simulink model "HighwayLaneChangePlanner"  (R2024b)
settings: Solver=FixedStepAuto  StartTime=0.0  StopTime=10.0  RelTol=1e-3  EnableMultiTasking=on
undefined symbols (not defined in the file or in its folder): actorProfiles, Ts
(part 1 of 2)
settings Model: Creator=The MathWorks, Inc.  LastModifiedBy=grape4314
settings SolverCC: AlgebraicLoopSolver=TrustRegion  MaxZcPerStep=1
settings DataIOCC: SaveOutput=off
settings OptimizationCC: DefaultParameterBehavior=Inlined  InlineInvariantSignals=on  EnhancedBackFolding=on  PassReuseOutputArgsAs=Individual arguments  ZeroExternalMemoryAtStartup=off  ZeroInternalMemoryAtStartup=off  EfficientFloat2IntCast=on  OptimizeBlockOrder=speed  DifferentSizesBufferReuse=on  OptimizationCustomize=off  EfficientTunableParamExpr=on
settings DebuggingCC: ParameterTunabilityLossMsg=error  UnconnectedInputMsg=warning  UnconnectedOutputMsg=warning  UnconnectedLineMsg=warning  ModelReferenceSymbolNameMessage=none  SubsystemReferenceDiagnosticForUnitTest=warning
settings HardwareCC: ProdLongLongMode=on
settings ModelReferenceCC: EnableRefExpFcnMdlSchedulingChecks=on  ModelReferenceNumInstancesAllowed=Single  PropagateVarSize=During execution
settings RTWCC: Description=Embedded Coder  SystemTargetFile=ert.tlc  TemplateMakefile=ert_default_tmf  RTWVerbose=off  BuildConfiguration=Faster Runs  PortableWordSizes=on  CodeExecutionProfiling=on  CodeProfilingSaveOptions=AllData  TargetLang=C++  GPUComputeCapability=3.5  DLArmComputeVersion=19.05
settings CodeAppCC: ForceParamTrailComments=on  IgnoreCustomStorageClasses=off  OperatorAnnotations=on  SimulinkDataObjDesc=on  SFDataObjDesc=on  CustomSymbolStrGlobalVar=$N$M  CustomSymbolStrType=$N$M_T  CustomSymbolStrFcn=APV_$N$M$F  CustomSymbolStrMacro=$N$M  InsertBlockDesc=on
settings ERTTargetCC: TargetLangStandard=C++03 (ISO)  GenerateSampleERTMain=on  CombineSignalStateStructs=on  CodeInterfacePackaging=C++ class  SupportVariableSizeSignals=on  RootIOFormat=Structure reference  ERTCustomFileTemplate=example_file_process.tlc  DynamicArrayContainerType=coder::array

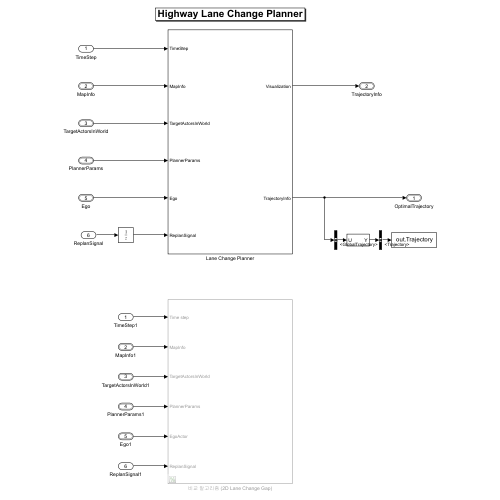
[thumbnail: Simulink's stored preview of the top-level diagram]
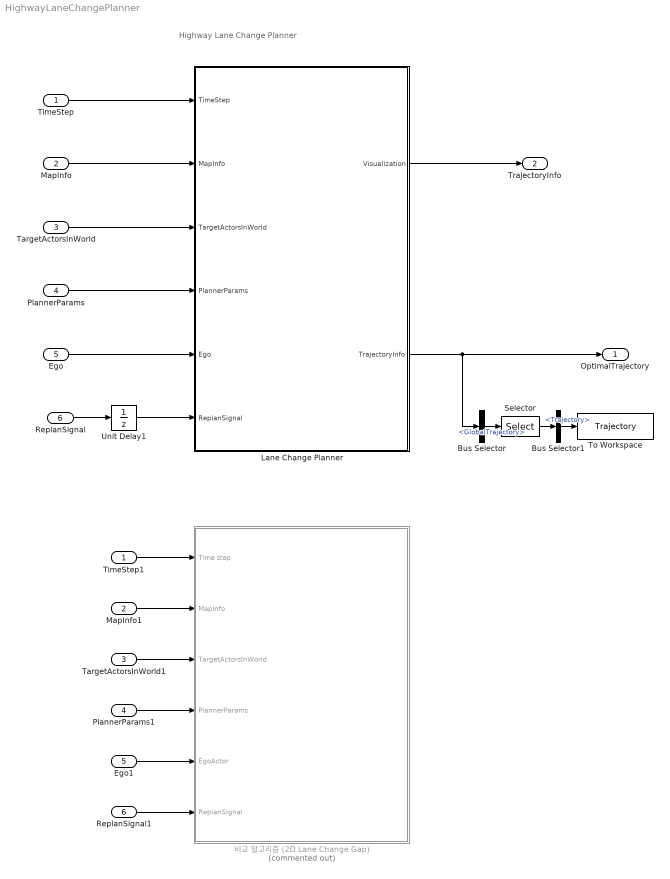
== system HighwayLaneChangePlanner ==
  note: Highway Lane Change Planner
  TimeStep : Inport
  MapInfo : Inport  Port=2  OutDataTypeStr=Bus: BusMapInfo  BusOutputAsStruct=on
  TargetActorsInWorld : Inport  Port=3  OutDataTypeStr=Bus: BusActorsEgo  BusOutputAsStruct=on
  PlannerParams : Inport  Port=4  OutDataTypeStr=Bus: BusPlannerParams  BusOutputAsStruct=on
  Ego : Inport  Port=5  OutDataTypeStr=Bus: BusVehiclePose
  ReplanSignal : Inport  Port=6
  Bus Selector : BusSelector  OutputSignals=GlobalTrajectory
  Bus Selector1 : BusSelector  OutputSignals=Trajectory
  Ego1 : InportShadow  Port=5  OutDataTypeStr=Bus: BusVehiclePose
  Lane Change Planner : Subsystem
  MapInfo1 : InportShadow  Port=2  OutDataTypeStr=Bus: BusMapInfo  BusOutputAsStruct=on
  PlannerParams1 : InportShadow  Port=4  OutDataTypeStr=Bus: BusPlannerParams  BusOutputAsStruct=on
  ReplanSignal1 : InportShadow  Port=6
  Selector : Selector  InputPortWidth=30  IndexOptions=Index vector (dialog)  Indices=1  OutputSizes=1
  TargetActorsInWorld1 : InportShadow  Port=3  OutDataTypeStr=Bus: BusActorsEgo  BusOutputAsStruct=on
  TimeStep1 : InportShadow
  To Workspace : ToWorkspace  VariableName=Trajectory  SaveFormat=Structure With Time  SampleTime=-1
  Unit Delay1 : UnitDelay  InitialCondition=1  SampleTime=-1  HasFrameUpgradeWarning=on
  비교 알고리즘 (2D Lane Change Gap) : Subsystem  Commented=on
  OptimalTrajectory : Outport  OutDataTypeStr=Bus: BusGlobalTrajectories  BusOutputAsStruct=on
  TrajectoryInfo : Outport  Port=2  OutDataTypeStr=Bus: BusVisualizationInfo  BusOutputAsStruct=on
  wires:
  TimeStep/1 -> Lane Change Planner/1(TimeStep)
  MapInfo/1 -> Lane Change Planner/2(MapInfo)
  TargetActorsInWorld/1 -> Lane Change Planner/3(TargetActorsInWorld)
  PlannerParams/1 -> Lane Change Planner/4(PlannerParams)
  Ego/1 -> Lane Change Planner/5(Ego)
  Lane Change Planner/1(Visualization) -> TrajectoryInfo/1
  Lane Change Planner/2(TrajectoryInfo) -> Bus Selector/1, OptimalTrajectory/1
  ReplanSignal/1 -> Unit Delay1/1
  Unit Delay1/1 -> Lane Change Planner/6(ReplanSignal)
  TimeStep1/1 -> 비교 알고리즘 (2D Lane Change Gap)/1(Time step)
  MapInfo1/1 -> 비교 알고리즘 (2D Lane Change Gap)/2(MapInfo)
  TargetActorsInWorld1/1 -> 비교 알고리즘 (2D Lane Change Gap)/3(TargetActorsInWorld)
  PlannerParams1/1 -> 비교 알고리즘 (2D Lane Change Gap)/4(PlannerParams)
  Ego1/1 -> 비교 알고리즘 (2D Lane Change Gap)/5(EgoActor)
  ReplanSignal1/1 -> 비교 알고리즘 (2D Lane Change Gap)/6(ReplanSignal)
  Bus Selector/1 -> Selector/1  "<GlobalTrajectory>"
  Bus Selector1/1 -> To Workspace/1  "<Trajectory>"
  Selector/1 -> Bus Selector1/1

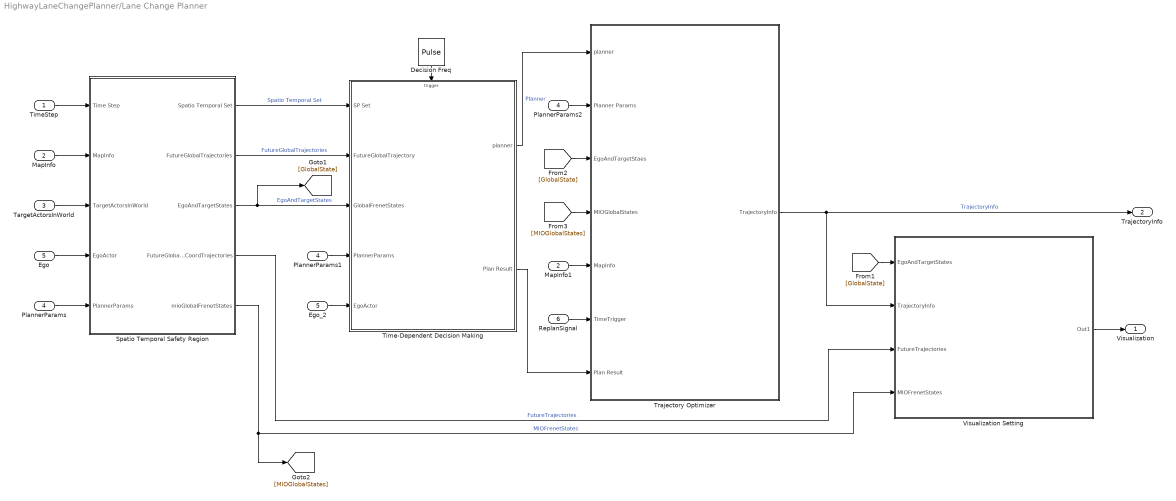
== system HighwayLaneChangePlanner/Lane Change Planner ==
  TimeStep : Inport
  MapInfo : Inport  Port=2  OutDataTypeStr=Bus: BusMapInfo  BusOutputAsStruct=on
  TargetActorsInWorld : Inport  Port=3  OutDataTypeStr=Bus: BusActorsEgo  BusOutputAsStruct=on
  PlannerParams : Inport  Port=4  OutDataTypeStr=Bus: BusPlannerParams  BusOutputAsStruct=on
  Ego : Inport  Port=5  OutDataTypeStr=Bus: BusVehiclePose
  ReplanSignal : Inport  Port=6
  Decision Freq : DiscretePulseGenerator  Period=10  SampleTime=Ts
  Ego_2 : InportShadow  Port=5  OutDataTypeStr=Bus: BusVehiclePose
  MapInfo1 : InportShadow  Port=2  OutDataTypeStr=Bus: BusMapInfo  BusOutputAsStruct=on
  PlannerParams1 : InportShadow  Port=4  OutDataTypeStr=Bus: BusPlannerParams  BusOutputAsStruct=on
  PlannerParams2 : InportShadow  Port=4  OutDataTypeStr=Bus: BusPlannerParams  BusOutputAsStruct=on
  Spatio Temporal Safety Region : Subsystem
  Time-Dependent Decision Making : Subsystem
  Trajectory Optimizer : Subsystem
  Visualization Setting : Subsystem
  Visualization : Outport  OutDataTypeStr=Bus: BusVisualizationInfo  BusOutputAsStruct=on
  TrajectoryInfo : Outport  Port=2  OutDataTypeStr=Bus: BusGlobalTrajectories
  wires:
  Spatio Temporal Safety Region/3(EgoAndTargetStates) -> Time-Dependent Decision Making/3(GlobalFrenetStates), [GlobalState]  "EgoAndTargetStates"
  Spatio Temporal Safety Region/1(Spatio Temporal Set) -> Time-Dependent Decision Making/1(SP Set)  "Spatio Temporal Set"
  Ego/1 -> Spatio Temporal Safety Region/4(EgoActor)
  Spatio Temporal Safety Region/2(FutureGlobalTrajectories) -> Time-Dependent Decision Making/2(FutureGlobalTrajectory)  "FutureGlobalTrajectories"
  PlannerParams/1 -> Spatio Temporal Safety Region/5(PlannerParams)
  TimeStep/1 -> Spatio Temporal Safety Region/1(Time Step)
  TargetActorsInWorld/1 -> Spatio Temporal Safety Region/3(TargetActorsInWorld)
  MapInfo/1 -> Spatio Temporal Safety Region/2(MapInfo)
  Ego_2/1 -> Time-Dependent Decision Making/5(EgoActor)
  Spatio Temporal Safety Region/4(FutureGlobalCoordTrajectories) -> Visualization Setting/3(FutureTrajectories)  "FutureTrajectories"
  Spatio Temporal Safety Region/5(mioGlobalFrenetStates) -> [MIOGlobalStates], Visualization Setting/4(MIOFrenetStates)  "MIOFrenetStates"
  Visualization Setting/1(Out1) -> Visualization/1
  [GlobalState] -> Visualization Setting/1(EgoAndTargetStates)
  PlannerParams1/1 -> Time-Dependent Decision Making/4(PlannerParams)
  Time-Dependent Decision Making/1(planner) -> Trajectory Optimizer/1(planner)  "Planner"
  PlannerParams2/1 -> Trajectory Optimizer/2(Planner Params)
  Time-Dependent Decision Making/2(Plan Result) -> Trajectory Optimizer/7(Plan Result)
  [GlobalState] -> Trajectory Optimizer/3(EgoAndTargetStaes)
  [MIOGlobalStates] -> Trajectory Optimizer/4(MIOGlobalStates)
  MapInfo1/1 -> Trajectory Optimizer/5(MapInfo)
  Trajectory Optimizer/1(TrajectoryInfo) -> TrajectoryInfo/1, Visualization Setting/2(TrajectoryInfo)  "TrajectoryInfo"
  ReplanSignal/1 -> Trajectory Optimizer/6(TimeTrigger)
  Decision Freq/1 -> Time-Dependent Decision Making/Trigger

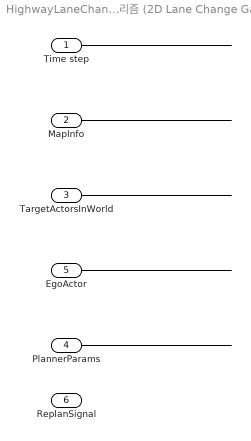
== system HighwayLaneChangePlanner/비교 알고리즘 (2D Lane Change Gap) ==
  Time step : Inport
  MapInfo : Inport  Port=2
  TargetActorsInWorld : Inport  Port=3
  PlannerParams : Inport  Port=4
  EgoActor : Inport  Port=5
  ReplanSignal : Inport  Port=6
  wires:
  Time step/1 -> ?
  MapInfo/1 -> ?
  TargetActorsInWorld/1 -> ?
  PlannerParams/1 -> ?
  EgoActor/1 -> ?

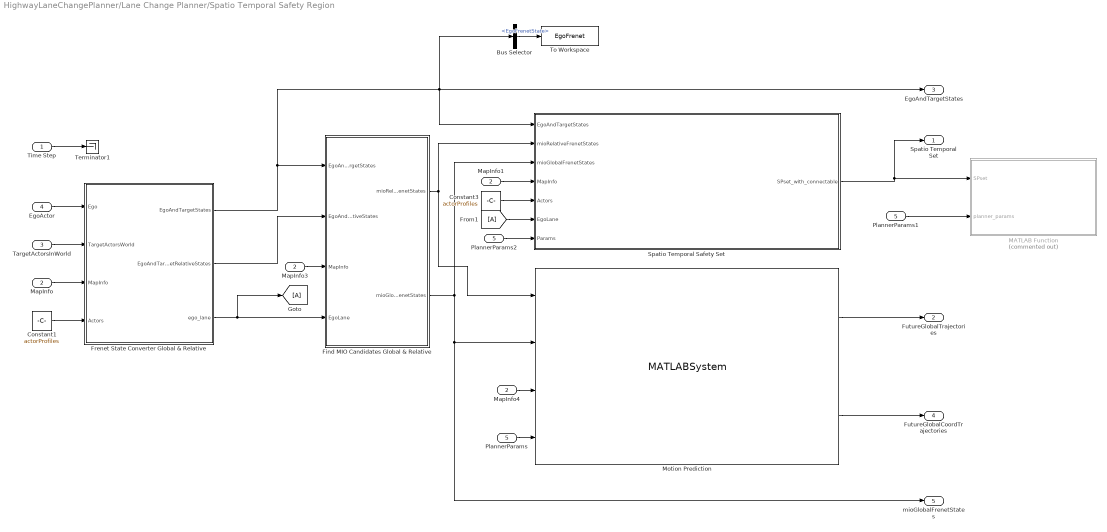
== system HighwayLaneChangePlanner/Lane Change Planner/Spatio Temporal Safety Region ==
  Time Step : Inport
  MapInfo : Inport  Port=2  OutDataTypeStr=Bus: BusMapInfo
  TargetActorsInWorld : Inport  Port=3  OutDataTypeStr=Bus: BusActorsEgo
  EgoActor : Inport  Port=4  OutDataTypeStr=Bus: BusVehiclePose
  PlannerParams : Inport  Port=5  OutDataTypeStr=Bus: BusPlannerParams
  Bus Selector : BusSelector  OutputSignals=EgoFrenetState
  Constant1 : Constant  Value=actorProfiles  OutDataTypeStr=Bus: BusActorProfiles
  Constant3 : Constant  Value=actorProfiles  OutDataTypeStr=Bus: BusActorProfiles
  Find MIO Candidates Global & Relative : MATLAB Function  TreatAsAtomicUnit=on
  Frenet State Converter Global & Relative : MATLAB Function  TreatAsAtomicUnit=on
  From1 : From
  Goto : Goto
  MATLAB Function : MATLAB Function  Commented=on  TreatAsAtomicUnit=on
  MapInfo1 : InportShadow  Port=2  OutDataTypeStr=Bus: BusMapInfo
  MapInfo3 : InportShadow  Port=2  OutDataTypeStr=Bus: BusMapInfo
  MapInfo4 : InportShadow  Port=2  OutDataTypeStr=Bus: BusMapInfo
  Motion Prediction : MATLABSystem  System=HelperMotionPrediction_RMC  SimulateUsing=Interpreted execution
      mask Type: HelperMotionPrediction_RMC
      mask Display:
      | disp('HelperMotionPrediction_RMC');
      | port_label('input',1,'MIOs_Relative');
      | port_label('input',2,'MIOs_Global');
      | port_label('input',3,'MapInfo');
      | port_label('input',4,'Params');
      | port_label('output',1,'FutureGlobalTrajectories');
      | port_label('output',2,'FutureGlobalCoordTrajectories');
  PlannerParams1 : InportShadow  Port=5  OutDataTypeStr=Bus: BusPlannerParams
  PlannerParams2 : InportShadow  Port=5  OutDataTypeStr=Bus: BusPlannerParams
  Spatio Temporal Safety Set : MATLAB Function  TreatAsAtomicUnit=on
  Terminator1 : Terminator
  To Workspace : ToWorkspace  VariableName=EgoFrenet  SaveFormat=Structure With Time  SampleTime=-1
  Spatio Temporal Set : Outport  OutDataTypeStr=Bus: BusSpatioTemporalSafetySet
  FutureGlobalTrajectories : Outport  Port=2  OutDataTypeStr=Bus: BusPredictedTrajectories
  EgoAndTargetStates : Outport  Port=3  OutDataTypeStr=Bus: BusEgoAndTargetStates
  FutureGlobalCoordTrajectories : Outport  Port=4
  mioGlobalFrenetStates : Outport  Port=5  OutDataTypeStr=Bus: BusMIOFrenetStates
  wires:
  Frenet State Converter Global & Relative/1(EgoAndTargetStates) -> Bus Selector/1, Spatio Temporal Safety Set/1(EgoAndTargetStates), EgoAndTargetStates/1, Find MIO Candidates Global & Relative/1(EgoAndTargetStates)
  Time Step/1 -> Terminator1/1
  EgoActor/1 -> Frenet State Converter Global & Relative/1(Ego)
  TargetActorsInWorld/1 -> Frenet State Converter Global & Relative/2(TargetActorsWorld)
  MapInfo/1 -> Frenet State Converter Global & Relative/3(MapInfo)
  Frenet State Converter Global & Relative/2(EgoAndTargetRelativeStates) -> Find MIO Candidates Global & Relative/2(EgoAndTargetRelativeStates)
  MapInfo3/1 -> Find MIO Candidates Global & Relative/3(MapInfo)
  Find MIO Candidates Global & Relative/1(mioRelativeFrenetStates) -> Motion Prediction/1, Spatio Temporal Safety Set/2(mioRelativeFrenetStates)
  MapInfo4/1 -> Motion Prediction/3
  PlannerParams/1 -> Motion Prediction/4
  Find MIO Candidates Global & Relative/2(mioGlobalFrenetStates) -> Spatio Temporal Safety Set/3(mioGlobalFrenetStates), mioGlobalFrenetStates/1, Motion Prediction/2
  Motion Prediction/2 -> FutureGlobalCoordTrajectories/1
  Constant1/1 -> Frenet State Converter Global & Relative/4(Actors)
  Frenet State Converter Global & Relative/3(ego_lane) -> Goto/1, Find MIO Candidates Global & Relative/4(EgoLane)
  Motion Prediction/1 -> FutureGlobalTrajectories/1
  From1/1 -> Spatio Temporal Safety Set/6(EgoLane)
  Constant3/1 -> Spatio Temporal Safety Set/5(Actors)
  MapInfo1/1 -> Spatio Temporal Safety Set/4(MapInfo)
  Spatio Temporal Safety Set/1(SPset_with_connectable) -> MATLAB Function/1(SPset), Spatio Temporal Set/1
  PlannerParams1/1 -> MATLAB Function/2(planner_params)
  PlannerParams2/1 -> Spatio Temporal Safety Set/7(Params)
  Bus Selector/1 -> To Workspace/1  "<EgoFrenetState>"

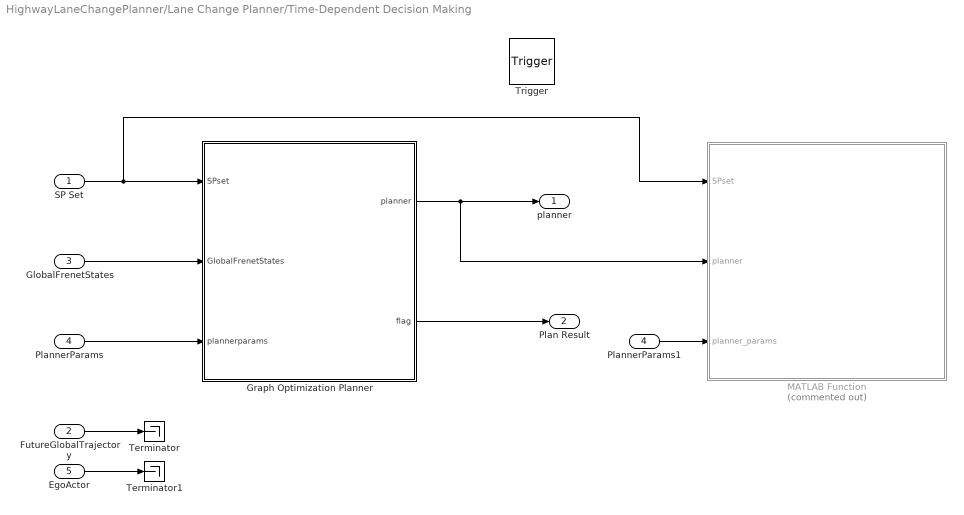
== system HighwayLaneChangePlanner/Lane Change Planner/Time-Dependent Decision Making ==
  SP Set : Inport  OutDataTypeStr=Bus: BusSpatioTemporalSafetySet
  FutureGlobalTrajectory : Inport  Port=2
  GlobalFrenetStates : Inport  Port=3  OutDataTypeStr=Bus: BusEgoAndTargetStates
  PlannerParams : Inport  Port=4  OutDataTypeStr=Bus: BusPlannerParams
  EgoActor : Inport  Port=5
  Trigger : TriggerPort  VariantControl=(inherit)  InitialTriggerSignalState=zero  PortDimensions=1
  Graph Optimization Planner : MATLAB Function  TreatAsAtomicUnit=on
  MATLAB Function : MATLAB Function  Commented=on  TreatAsAtomicUnit=on
  PlannerParams1 : InportShadow  Port=4  OutDataTypeStr=Bus: BusPlannerParams
  Terminator : Terminator
  Terminator1 : Terminator
  planner : Outport  OutDataTypeStr=Bus: BusGraphPlanner
  Plan Result : Outport  Port=2
  wires:
  FutureGlobalTrajectory/1 -> Terminator/1
  GlobalFrenetStates/1 -> Graph Optimization Planner/2(GlobalFrenetStates)
  EgoActor/1 -> Terminator1/1
  SP Set/1 -> MATLAB Function/1(SPset), Graph Optimization Planner/1(SPset)
  PlannerParams/1 -> Graph Optimization Planner/3(plannerparams)
  Graph Optimization Planner/1(planner) -> MATLAB Function/2(planner), planner/1
  Graph Optimization Planner/2(flag) -> Plan Result/1
  PlannerParams1/1 -> MATLAB Function/3(planner_params)

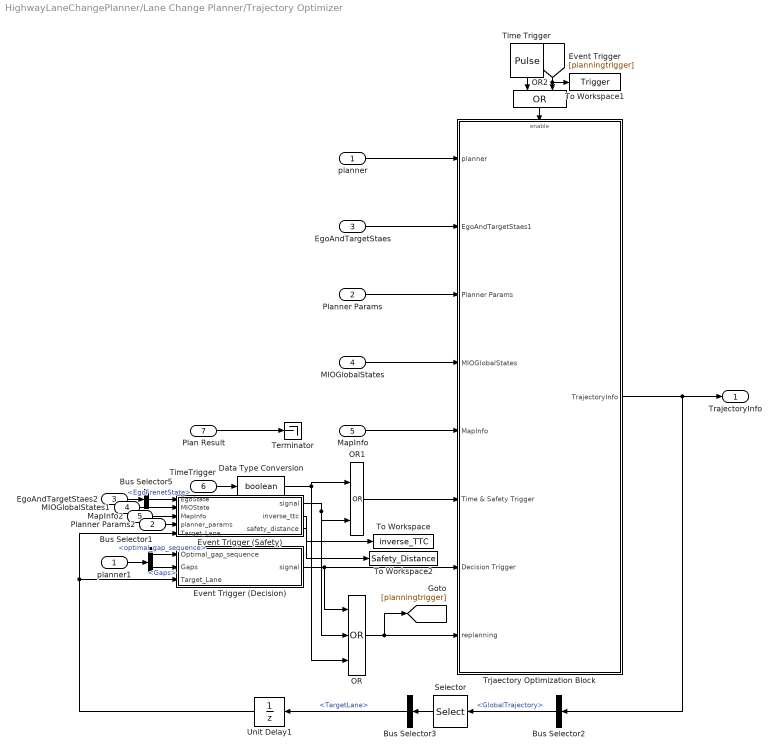
== system HighwayLaneChangePlanner/Lane Change Planner/Trajectory Optimizer ==
  planner : Inport  OutDataTypeStr=Bus: BusGraphPlanner
  Planner Params : Inport  Port=2  OutDataTypeStr=Bus: BusPlannerParams
  EgoAndTargetStaes : Inport  Port=3
  MIOGlobalStates : Inport  Port=4
  MapInfo : Inport  Port=5  OutDataTypeStr=Bus: BusMapInfo
  TimeTrigger : Inport  Port=6
  Plan Result : Inport  Port=7
  Bus Selector1 : BusSelector  OutputSignals=optimal_gap_sequence,Gaps
  Bus Selector2 : BusSelector  OutputSignals=GlobalTrajectory
  Bus Selector3 : BusSelector  OutputSignals=TargetLane
  Bus Selector5 : BusSelector  OutputSignals=EgoFrenetState
  Data Type Conversion : DataTypeConversion  OutDataTypeStr=boolean  SaturateOnIntegerOverflow=off  RndMeth=Floor
  EgoAndTargetStaes2 : InportShadow  Port=3
  Event Trigger (Decision) : MATLAB Function  TreatAsAtomicUnit=on
  Event Trigger (Safety) : MATLAB Function  TreatAsAtomicUnit=on
  MIOGlobalStates1 : InportShadow  Port=4
  MapInfo2 : InportShadow  Port=5  OutDataTypeStr=Bus: BusMapInfo
  OR : Logic  Operator=OR  Inputs=3  IconShape=distinctive  AllPortsSameDT=off  OutDataTypeStr=boolean
  OR1 : Logic  Operator=OR  IconShape=distinctive  AllPortsSameDT=off  OutDataTypeStr=boolean
  OR2 : Logic  Operator=OR  IconShape=distinctive  AllPortsSameDT=off  OutDataTypeStr=boolean
  Planner Params2 : InportShadow  Port=2  OutDataTypeStr=Bus: BusPlannerParams
  Selector : Selector  InputPortWidth=30  IndexOptions=Index vector (dialog)  Indices=1  OutputSizes=1
  Terminator : Terminator
  Time Trigger : DiscretePulseGenerator  Period=5  SampleTime=Ts
  To Workspace : ToWorkspace  VariableName=inverse_TTC  SaveFormat=Structure With Time  SampleTime=-1
  To Workspace1 : ToWorkspace  VariableName=Trigger  SaveFormat=Structure With Time  SampleTime=-1
  To Workspace2 : ToWorkspace  VariableName=Safety_Distance  SaveFormat=Structure With Time  SampleTime=-1
  Trjaectory Optimization Block : Subsystem
  Unit Delay1 : UnitDelay  SampleTime=-1  HasFrameUpgradeWarning=on
  planner1 : InportShadow  OutDataTypeStr=Bus: BusGraphPlanner
  TrajectoryInfo : Outport  OutDataTypeStr=Bus: BusGlobalTrajectories
  wires:
  EgoAndTargetStaes2/1 -> Bus Selector5/1
  planner/1 -> Trjaectory Optimization Block/1(planner)
  Bus Selector5/1 -> Event Trigger (Safety)/1(EgoState)  "<EgoFrenetState>"
  Event Trigger (Decision)/1(signal) -> Trjaectory Optimization Block/7(Decision Trigger), OR/1
  Plan Result/1 -> Terminator/1
  TimeTrigger/1 -> Data Type Conversion/1
  MIOGlobalStates1/1 -> Event Trigger (Safety)/2(MIOState)
  MapInfo2/1 -> Event Trigger (Safety)/3(MapInfo)
  EgoAndTargetStaes/1 -> Trjaectory Optimization Block/2(EgoAndTargetStaes1)
  Planner Params/1 -> Trjaectory Optimization Block/3(Planner Params)
  Trjaectory Optimization Block/1(TrajectoryInfo) -> Bus Selector2/1, TrajectoryInfo/1
  MIOGlobalStates/1 -> Trjaectory Optimization Block/4(MIOGlobalStates)
  MapInfo/1 -> Trjaectory Optimization Block/5(MapInfo)
  Bus Selector1/1 -> Event Trigger (Decision)/1(Optimal_gap_sequence)  "<optimal_gap_sequence>"
  Bus Selector1/2 -> Event Trigger (Decision)/2(Gaps)  "<Gaps>"
  planner1/1 -> Bus Selector1/1
  Data Type Conversion/1 -> OR1/1, OR/3
  OR1/1 -> Trjaectory Optimization Block/6(Time & Safety Trigger)
  Event Trigger (Safety)/1(signal) -> OR/2, OR1/2
  OR/1 -> [planningtrigger], Trjaectory Optimization Block/8(replanning)
  Bus Selector3/1 -> Unit Delay1/1  "<TargetLane>"
  Selector/1 -> Bus Selector3/1
  Bus Selector2/1 -> Selector/1  "<GlobalTrajectory>"
  Unit Delay1/1 -> Event Trigger (Decision)/3(Target_Lane), Event Trigger (Safety)/5(Target_Lane)
  OR2/1 -> Trjaectory Optimization Block/Enable
  Time Trigger/1 -> OR2/1
  [planningtrigger] -> To Workspace1/1, OR2/2
  Planner Params2/1 -> Event Trigger (Safety)/4(planner_params)
  Event Trigger (Safety)/2(inverse_ttc) -> To Workspace/1
  Event Trigger (Safety)/3(safety_distance) -> To Workspace2/1

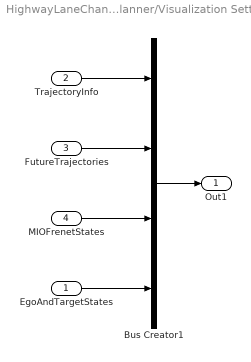
== system HighwayLaneChangePlanner/Lane Change Planner/Visualization Setting ==
  EgoAndTargetStates : Inport
  TrajectoryInfo : Inport  Port=2
  FutureTrajectories : Inport  Port=3
  MIOFrenetStates : Inport  Port=4
  Bus Creator1 : BusCreator  Inputs=4  OutDataTypeStr=Bus: BusVisualizationInfo
  Out1 : Outport  OutDataTypeStr=Bus: BusVisualizationInfo
  wires:
  Bus Creator1/1 -> Out1/1
  FutureTrajectories/1 -> Bus Creator1/2
  TrajectoryInfo/1 -> Bus Creator1/1
  EgoAndTargetStates/1 -> Bus Creator1/4
  MIOFrenetStates/1 -> Bus Creator1/3

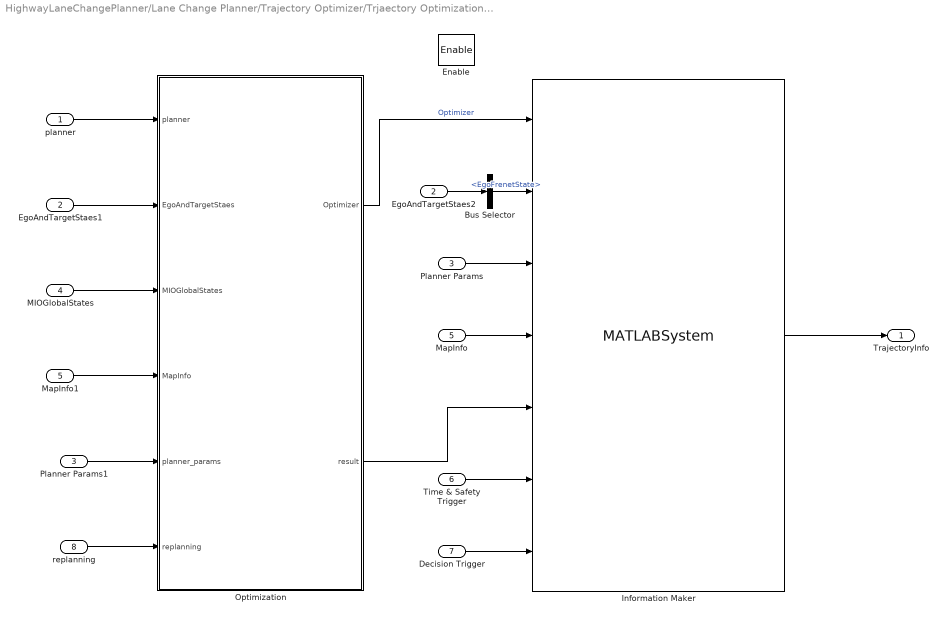
== system HighwayLaneChangePlanner/Lane Change Planner/Trajectory Optimizer/Trjaectory Optimization Block ==
  planner : Inport
  EgoAndTargetStaes1 : Inport  Port=2
  Planner Params : Inport  Port=3  OutDataTypeStr=Bus: BusPlannerParams
  MIOGlobalStates : Inport  Port=4
  MapInfo : Inport  Port=5  OutDataTypeStr=Bus: BusMapInfo
  Time & Safety Trigger : Inport  Port=6
  Decision Trigger : Inport  Port=7
  replanning : Inport  Port=8
  Enable : EnablePort
  Bus Selector : BusSelector  OutputSignals=EgoFrenetState
  EgoAndTargetStaes2 : InportShadow  Port=2
  Information Maker : MATLABSystem  System=HelperMakeTrajectory  SimulateUsing=Interpreted execution
      mask Type: HelperMakeTrajectory
      mask Display:
      | disp('HelperMakeTrajectory');
      | port_label('input',1,'Optimizer');
      | port_label('input',2,'EgoState');
      | port_label('input',3,'params');
      | port_label('input',4,'MapInfo');
      | port_label('input',5,'Planresult');
      | port_label('input',6,'replanningSignal');
      | port_label('input',7,'resamplingSignal');
      | port_label('output',1,'GlobalTrajectories');
  MapInfo1 : InportShadow  Port=5  OutDataTypeStr=Bus: BusMapInfo
  Optimization : MATLAB Function  TreatAsAtomicUnit=on
  Planner Params1 : InportShadow  Port=3  OutDataTypeStr=Bus: BusPlannerParams
  TrajectoryInfo : Outport
  wires:
  Bus Selector/1 -> Information Maker/2  "<EgoFrenetState>"
  Optimization/2(result) -> Information Maker/5
  Time & Safety Trigger/1 -> Information Maker/6
  Optimization/1(Optimizer) -> Information Maker/1  "Optimizer"
  Information Maker/1 -> TrajectoryInfo/1
  EgoAndTargetStaes2/1 -> Bus Selector/1
  MapInfo/1 -> Information Maker/4
  replanning/1 -> Optimization/6(replanning)
  Planner Params/1 -> Information Maker/3
  planner/1 -> Optimization/1(planner)
  MapInfo1/1 -> Optimization/4(MapInfo)
  Decision Trigger/1 -> Information Maker/7
  EgoAndTargetStaes1/1 -> Optimization/2(EgoAndTargetStaes)
  MIOGlobalStates/1 -> Optimization/3(MIOGlobalStates)
  Planner Params1/1 -> Optimization/5(planner_params)

== matlab function HighwayLaneChangePlanner/Lane Change Planner/Spatio Temporal Safety Region/Find MIO Candidates Global & Relative ==
  data: EgoAndTargetStates input; EgoAndTargetRelativeStates input; MapInfo input; mioRelativeFrenetStates output Bus: BusMIOFrenetStates; mioGlobalFrenetStates output Bus: BusMIOFrenetStates; EgoLane input
function [mioRelativeFrenetStates,mioGlobalFrenetStates] =  findMIOs(EgoAndTargetStates,...
                                                                     EgoAndTargetRelativeStates,...
                                                                     MapInfo, EgoLane)

%%% EgoAndTargetRelativeState %%%
%%% 1. NumTargetActors      : 총 주변 차량 수
%%% 2. TargetRelativeStates : 주변 차량의 RelativeStates with respect to World Coordinate(x, y, Yaw, Kappa, Velocity, accel)
%%% 3. TargetFrenetStates   : 주변 차량의 RelativeStates with respect to Frenet States (s, ds, dds, l, dl, ddl)
%%% 4. TargetIDs            : 주변 차량의 고유번호
%%% 5. EgoGlobalFrenetState : Ego 차량의 Frenet States

coder.inline('never');
%findMIOs function block identifies Most Importent Objects(MIOs) in the
%scenario.


% Get the number of target actors in the scenario from EgoAndTargetStates
numTargets = EgoAndTargetRelativeStates.NumTargetActors;

% Get target actors frenet states from EgoAndTargetStates bus structure.
targetRelativeFrenetStates = EgoAndTargetRelativeStates.TargetRelativeFrenetStates;
targetGlobalFrenetStates = EgoAndTargetStates.TargetFrenetStates;
targetIDs = EgoAndTargetRelativeStates.TargetIDs;

% Get ego actor frenet states from EgoAndTargetStates bus structure
egoFrenetState = EgoAndTargetRelativeStates.EgoGlobalFrenetState;

% Invoke the wrapper function helperFindMIOs
% {NumMios, LaneNumbers, TTc, RelativeDist, RelativeVel, Issafe, Isfront}
initStruct = HelperLCPlannerDefaultData.MIOFrenetStates;
mioRelativeFrenetStates = initStruct;
mioGlobalFrenetStates = initStruct;

% Invoke the wrapper function to get the MIOs Info
if(numTargets)
    [mioRelativeFrenetStates,...
     mioGlobalFrenetStates] =  helperFindMIOCandidates_RMC(egoFrenetState,...
                                                           MapInfo,...
                                                           targetRelativeFrenetStates(1:numTargets,:),...
                                                           targetGlobalFrenetStates(1:numTargets,:),...
                                                           targetIDs(1:numTargets,:), EgoLane, ...
                                                           initStruct);
end

end

== matlab function HighwayLaneChangePlanner/Lane Change Planner/Trajectory Optimizer/Event Trigger (Safety) ==
  data: EgoState input; MIOState input; MapInfo input; signal output; planner_params input; Target_Lane input; inverse_ttc output; safety_distance output
function [signal, inverse_ttc, safety_distance] = safety_trigger(EgoState, MIOState, MapInfo, planner_params, Target_Lane)

    persistent prev_result

    if isempty(prev_result)
        prev_result = false;
    end
 

    if Target_Lane == 0
        % 초기화
        inverse_ttc = 0;
        signal = false;
        ttc = planner_params.MaxTTC;
        safety_distance = 150;
        return;
    end

    signal = false;
    ttc_vio = false;
    Target_lane_center = MapInfo.LaneCenters(Target_Lane);
    Target_MIO_State = select_target_mio(Target_lane_center, EgoState, MIOState, MapInfo);
    MaxTTC = planner_params.MaxTTC;
    MinTTC = planner_params.MinTTC;
    MaxFront = planner_params.MaxFront;
    MaxRear = planner_params.MaxRear;

    if all(Target_MIO_State == 0)
        % MIO Detection이 안되는 경우 (매우 안전)
        ttc = MaxTTC;
        inverse_ttc = 0;
        safety_distance = 150;
        signal = false;
        prev_result = signal;
        return;
    end

    if Target_MIO_State(1) > EgoState(1) && Target_MIO_State(2) < EgoState(2)
        % 전방 MIO에 대해 TTC 정의되는 경우
        Delta_s = Target_MIO_State(1) - EgoState(1);
        Delta_v = (EgoState(2)-Target_MIO_State(2));

        if Delta_s - MaxFront <= 0
            % 안전 위배
            ttc = 0;
        else
            ttc = (Delta_s - MaxFront) / Delta_v;
        end

        inverse_ttc = Delta_v / max(0.001, Delta_s - MaxFront);
        % inverse_ttc = min(1/MinTTC, inverse_ttc);

        if ttc < MinTTC
            ttc_vio = true;
        end
    elseif Target_MIO_State(1) < EgoState(1) && Target_MIO_State(2) > EgoState(2)
        % 후방 MIO에 대해 TTC 정의되는 경우
        Delta_s = EgoState(1) - Target_MIO_State(1);
        Delta_v = Target_MIO_State(2) - EgoState(2);

        if Delta_s - MaxRear <= 0
            % 안전 위배
            ttc = 0;
        else
            ttc = (Delta_s - MaxRear) / Delta_v;
        end

        inverse_ttc = Delta_v / max(0.001, Delta_s - MaxRear);
        % inverse_ttc = min(1/MinTTC, inverse_ttc);

        if ttc < MinTTC
            ttc_vio = true;
        end
    else
        % TTC 정의가 안되는 경우 (매우 안전)
        %   1. 전방 차량이 더 빠름
        %   2. 후방 차량이 더 느림
        ttc = MaxTTC;
        inverse_ttc = 0;
    end

    safety_distance = abs(Target_MIO_State(1) - EgoState(1));

    if ttc_vio && ~prev_result
        signal = true;
        prev_result = signal;
    elseif ttc_vio && prev_result
        signal = false;
    elseif ~ttc_vio
        signal = false;
        prev_result = signal;
    end
    signal = false;
end

function Target_MIO_State = select_target_mio(Target_lane_center, EgoState, MIOState, MapInfo)
    NumMIOs = MIOState.NumMIOs;
    MIOStates = MIOState.MIOStates;
    LaneWidth = MapInfo.LaneWidth(1);
    Target_MIO_State = zeros(1, 6);
    % Target으로 잡아야 하는 MIO 선정
    if NumMIOs > 0
        Target_d = Target_lane_center;
        MIO_d_e = MIOStates(1:NumMIOs, 4) - Target_d;
        valid_MIO_ids = find(abs(MIO_d_e) <= LaneWidth/2);
        if ~isempty(valid_MIO_ids)
            % Valid MIO가 존재하는 경우
            valid_MIOState = MIOStates(valid_MIO_ids, :); % (n, 6)
            if size(valid_MIOState, 1) > 1
                % Valid MIO가 2대 이상인 경우, 제일 가까운 MIO로 선정
                [~, target_ids] = min(abs(valid_MIOState(:, 1) - EgoState(1)));
                target_MIOState = valid_MIOState(target_ids, :);
            else
                % Valid MIO가 1대인 경우
                target_MIOState = valid_MIOState(1, :);
            end
            Target_MIO_State(:) = target_MIOState;
        end 
    end
end

== matlab function HighwayLaneChangePlanner/Lane Change Planner/Spatio Temporal Safety Region/Spatio Temporal Safety Set ==
  data: EgoAndTargetStates input; mioRelativeFrenetStates input; SPset_with_connectable output Bus: BusSpatioTemporalSafetySet; mioGlobalFrenetStates input; MapInfo input; Actors input; EgoLane input; Params input
function SPset_with_connectable = SpatioTemporalSafetySet(EgoAndTargetStates, mioRelativeFrenetStates, mioGlobalFrenetStates, MapInfo, Actors, EgoLane, Params)

%%% mioRelativeFrenetStates %%%
%%% 1. NumMIOs      : MIO 개수
%%% 2. TargetIds    : MIO 차량들의 고유번호
%%% 3. MIOStates    : MIO 차량들의 Frenet States (s ds dds l dl ddl)

%%% mioGlobalFrenetStates %%%
%%% 1. NumMIOs      : MIO 개수
%%% 2. TargetIds    : MIO 차량들의 고유번호
%%% 3. MIOStates    : MIO 차량들의 Frenet States (s ds dds l dl ddl)

%%% FutureGlobalTrajectory %%%
%%% 1. NumTrajs     : Trajectroy 개수 (= MIO 개수)
%%% 2. TargetIDs    : MIO 고유번호
%%% 3. Trajectories : Trajectory 객체 (TargetID, NumPts, Trajectory)

%%% MapInfo %%%
%%% 1. NumLanes             : 차선 개수
%%% 2. LaneWidth            : 차선 폭
%%% 3. LaneCenter           : 차선 중심
%%% 4. NumGlobalPlanPoints  : Global Waypoint 개수
%%% 5. GlobalPlanPoints     : Global Waypoint 초기경로
%%% 6. LaneLateralBoundary  : 차선의 횡방향 Boundary

initStruct = HelperLCPlannerDefaultData.SpatioTemporalSafetySet;
initStruct_LC = HelperLCPlannerDefaultData.LCConnectableSet;
initStruct_LK = HelperLCPlannerDefaultData.LKConnectableSet;
EgoActor = Actors(1);
EgoState = EgoAndTargetStates.EgoFrenetState;

SpatioTemporalSet = helperCreateSpatioTemporalSafetySet_Freeset(mioRelativeFrenetStates, ...
                                                                mioGlobalFrenetStates, ...
                                                                MapInfo, ...
                                                                initStruct, ...
                                                                EgoState, ...
                                                                EgoActor, ...
                                                                EgoLane, ...
                                                                Params);

SPset_with_connectable = helperCreateConnectableSet(initStruct_LC, ...
                                                    initStruct_LK, ...
                                                    SpatioTemporalSet);


end

== matlab function HighwayLaneChangePlanner/Lane Change Planner/Spatio Temporal Safety Region/MATLAB Function ==
  data: SPset input; planner_params input
function VisualDispatch(SPset, planner_params)
% C_now, T_now : "현재 프레임"의 Bus (누적 아님)
% trigger       : 논리. true일 때만 그림
% mode          : uint8(1=all, 2=spatio-only, 3=temporal-only, 4=opt-path)
% decim         : uint32, N스텝마다 1회만 그림
%#codegen

    persistent stepCnt decim
    if isempty(stepCnt) 
        stepCnt = 0;
        decim = 30;
    end

    C_now = SPset.Cc_t;
    T_now = SPset.Ck_t;
    planning_horizon = planner_params.TimeHorizon;
    planning_resolution = planner_params.PlanningResolution;
    ego = struct("x0", 0, "y0", 0);

    % 코드생성/Accelerator 경로에서는 아무 것도 하지 않음
    if coder.target('Rtw') || coder.target('MEX')
        return;
    end
    
    % extrinsic 선언 (Visualizer는 static 메서드)
    coder.extrinsic('Visualizer.visualize_all_connectivity_3D');
    coder.extrinsic('Visualizer.visualize_spatio_connectivity_3D');
    coder.extrinsic('Visualizer.visualize_temporal_connections_with_set');
    coder.extrinsic('Visualizer.setup_3D_plot_aesthetics');
    coder.extrinsic('Visualizer.highlight_optimal_path');
    
    if mod(stepCnt, decim) == 0
        Visualizer.visualize_all_connectivity_3D(C_now, T_now, planning_horizon, planning_resolution, 10.0, ego);
    end
    stepCnt = stepCnt + 1;
end

== matlab function HighwayLaneChangePlanner/Lane Change Planner/Time-Dependent Decision Making/MATLAB Function ==
  data: SPset input; planner input; planner_params input
function VisualDispatch(SPset, planner, planner_params)
    %#codegen
    persistent stepCnt decim
    if isempty(stepCnt) 
        stepCnt = 0;
        decim = 6;
    end

    C_now = SPset.Cc_t;
    T_now = SPset.Ck_t;
    ego = struct("x0", 0, "y0", 0);
    optimal_gap_sequence_ids = planner.optimal_gap_sequence;
    planning_horizon = planner_params.TimeHorizon;
    planning_resolution = planner_params.PlanningResolution;
    num_nodes = planner.num_total_nodes;
    adjacency_mtrx = planner.adjacency_matrix(1:num_nodes, 1:num_nodes);

    % 코드생성/Accelerator 경로에서는 아무 것도 하지 않음
    if coder.target('Rtw') || coder.target('MEX')
        return;
    end
    
    % extrinsic 선언 (Visualizer는 static 메서드)
    coder.extrinsic('isualizer.highlight_optimal_edges');
    coder.extrinsic('Visualizer.highlight_optimal_nodes');
    coder.extrinsic('Visualizer.highlight_optimal_path');
    coder.extrinsic('Visualizer.draw_node_costs');
    coder.extrinsic('Visualizer.visualize_all_connectivity_3D');
    coder.extrinsic('Visualizer.visualize_spatio_connectivity_3D');
    coder.extrinsic('Visualizer.visualize_temporal_connections_with_set');
    coder.extrinsic('Visualizer.setup_3D_plot_aesthetics');
    coder.extrinsic('Visualizer.highlight_optimal_path');
    coder.extrinsic('Visualizer.visualize');
    
    if mod(stepCnt, decim) == 0
        Visualizer.visualize(C_now, T_now, optimal_gap_sequence_ids, planning_horizon, planning_resolution, 10.0, ego, adjacency_mtrx);
    end
    stepCnt = stepCnt + 1;
end

== matlab function HighwayLaneChangePlanner/Lane Change Planner/Time-Dependent Decision Making/Graph Optimization Planner ==
  data: SPset input Bus: BusSpatioTemporalSafetySet; GlobalFrenetStates input; plannerparams input; planner output Bus: BusGraphPlanner; flag output
function [planner, flag] = plan(SPset, GlobalFrenetStates, plannerparams)

    lane_change_coeff = plannerparams.lane_change_coeff;
    change_difficulty_coeff = plannerparams.change_difficulty_coeff;


    LK_set = SPset.Ck_t;
    LC_set = SPset.Cc_t;
    EgoState = GlobalFrenetStates.EgoFrenetState;

    InitStruct = HelperLCPlannerDefaultData.GraphPlanner;
    
    max_id = 0;
    num_total_gaps = 0;
    %% 초기 데이터 세팅
    for i = 1:length(LC_set)
        cc_t = LC_set(i);
        num_gaps = cc_t.num_gaps;
        for j = 1:num_gaps
            gap = cc_t.gaps(j);
            if gap.idx > max_id
                max_id = gap.idx;
            end
            num_total_gaps = num_total_gaps + 1;
            InitStruct.Gaps(num_total_gaps) = gap;
        end
    end
    % Gap 정보를 global ID 기반 배열로 저장
    gap_lane_idx = zeros(max_id, 1);
    gap_s = zeros(max_id, 1);
    gap_d = zeros(max_id, 1);
    gap_l = zeros(max_id, 1);
    gap_time_idx = zeros(max_id, 1);
    
    node_costs = zeros(max_id, 1);
    for i = 1:num_total_gaps
        gap = InitStruct.Gaps(i);
        InitStruct.Gaps(i).node_cost = gap.node_cost;
        % Node 고유 비용 저장
        node_costs(gap.idx) = gap.node_cost;
        % Gap 정보 배열에 저장
        gap_lane_idx(gap.idx) = gap.lane_idx;
        gap_s(gap.idx) = gap.s;
        gap_d(gap.idx) = gap.d;
        gap_l(gap.idx) = gap.l;
        gap_time_idx(gap.idx) = gap.time_idx;
    end

    %% 엣지 리스트 세팅
    S_LC = zeros(max_id*(max_id-1)/2, 1);
    T_LC = zeros(max_id*(max_id-1)/2, 1);
    S_LK = zeros(max_id*(max_id-1)/2, 1);
    T_LK = zeros(max_id*(max_id-1)/2, 1);

    m_lc = 0; % LC 엣지 리스트 갯수
    for i = 1:length(LC_set)
        LC_graph = LC_set(i).spatio_topology_global_graph;
        num_nodes = LC_set(i).num_nodes; % 이번 스텝에서의 LC Connection Edge
        if ~isempty(LC_graph)
            S_LC(m_lc+1:m_lc+num_nodes) = LC_graph(1, 1:num_nodes);
            T_LC(m_lc+1:m_lc+num_nodes) = LC_graph(2, 1:num_nodes);
            m_lc = m_lc + num_nodes;
        end
    end

    m_lk = 0; % LK 엣지 리스트 갯수
    for i = 1:length(LK_set)
        LK_graph = LK_set(i).temporal_topology_global_graph;
        num_nodes = LK_set(i).num_nodes;
        if ~isempty(LK_graph)
            S_LK(m_lk+1:m_lk+num_nodes) = LK_graph(1, 1:num_nodes);
            T_LK(m_lk+1:m_lk+num_nodes) = LK_graph(2, 1:num_nodes);
            m_lk = m_lk + num_nodes;
        end
    end

    %% Adjacency Matrix 세팅
    adjacency_matrix = inf(max_id, max_id);
    
    for i = 1:m_lc
        source = S_LC(i);
        target = T_LC(i);

        source_s = gap_s(source);
        source_d = gap_d(source);
        target_s = gap_s(target);
        target_d = gap_d(target);
        source_gap_length = gap_l(source);
        target_gap_length = gap_l(target); 

        source_s_max = max(0, source_s + source_gap_length/2);
        source_s_min = max(0, source_s - source_gap_length/2);
        target_s_max = max(0, target_s + target_gap_length/2);
        target_s_min = max(0, target_s - target_gap_length/2);

        % 기본 lane change 비용
        lane_change = abs(source_d - target_d) / 3.6; % [0, 1] : LaneWidth=3.6
        
        % Lane Change 난이도 비용 (겹침 정도로 정량화)
        gap_overlap = min(source_s_max, target_s_max) - max(source_s_min, target_s_min);
        if gap_overlap > 0
            % Gap overlap이 증가할수록 난이도 하락 -> 비용 감소
            difficulty = max(0, (source_gap_length - gap_overlap) / source_gap_length);
        else
            % 겹침 정도가 0
            difficulty = inf;
        end

        transition_cost = 1.0 * lane_change_coeff * lane_change +...
                          1.0 * change_difficulty_coeff * difficulty;

        % transition_cost = 1.0 * lane_change_coeff * lane_change;

        adjacency_matrix(source, target) = transition_cost;
    end

    for i = 1:m_lk
        source = S_LK(i);
        target = T_LK(i);
        adjacency_matrix(source, target) = 0;
    end

    %% Start, End Nodes 세팅
    cc_t0 = LC_set(1);
    cc_tf = LC_set(end);
    x_ego = 0; % Position은 Ego 기준
    y_ego = 0; % Position은 Ego 기준 
    start_node = 1;
    end_nodes = [cc_tf.gaps(1:cc_tf.num_gaps)];
    end_nodes = [end_nodes.idx];
    for i = 1:cc_t0.num_gaps
        if y_ego == cc_t0.gaps(i).d
            if (x_ego >= cc_t0.gaps(i).s - cc_t0.gaps(i).l/2 ) && (x_ego <= cc_t0.gaps(i).s + cc_t0.gaps(i).l/2)
                start_node = cc_t0.gaps(i).idx;
                break;
            end
        end
    end

    
    %% Planner에 데이터 세팅
    InitStruct.adjacency_matrix(1:max_id, 1:max_id) = adjacency_matrix;
    InitStruct.num_total_nodes = max_id;

    if isempty(start_node) || isempty(end_nodes)
        planner = InitStruct;
        flag = false;
    else
        %% Dijkstra Graph Search
        num_end_nodes = length(end_nodes);
        InitStruct.start_node = start_node;
        InitStruct.end_nodes(1:num_end_nodes) = end_nodes;
        planner = helperFindoptimalsequence(InitStruct, ...
                                            node_costs, ...
                                            LK_set, ...
                                            LC_set, ...
                                            EgoState, ...
                                            plannerparams);
        flag = true;
    end
    
end
